simulink library "lib_Convection_LamIntFlwVarShapes"  (R2015a)
settings: Solver=ode45  StartTime=0.0  StopTime=10.0  RelTol=1e-3
libraries: simulink x5, lib_GenTools_MinMax x1
settings Model: Creator=jlkratz  LastModifiedBy=jlkratz

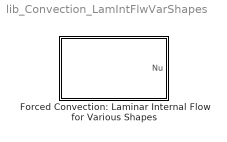
== system lib_Convection_LamIntFlwVarShapes ==
  Forced Convection: Laminar Internal Flow for Various Shapes : Subsystem  mask(TSAT: Laminar Flow for Various Shaped Tubes){Shape_M=Circle, IsothermOrIsoflux_M=Isothermal, FinOrInf_M=Finite Aspect Ratio, boa_M=1, HeatBothOrInsulateOne_M=Both sides heated}
      mask prompts: Shape_M "Shape_M - Cross-section shape"; IsothermOrIsoflux_M "IsothermOrIsoflux_M - Check for isothermal surfaces, unchecked for isoflux surfaces"; boa_M "boa_M - Aspect ratio of the rectangular cross-section (b/a) where b is the longer side"
      mask help:
      | This block provides the Nusselt number for fully developed laminar flow within tubes of different cross-sections. Options include circular, rectangular, and triangular cross-sections with isothermal and isoflux surfaces. In the case of rectangular flow paths the scenario of an infinite aspect ratio flow path is considered. This situation has options for when both sides of the flow path are heated and when one side is heated and the other is insulated. Note that when using the Nusselt number to calculate the convective heat transfer coefficient, the hydraulic diameter should be used.
      |
      | See the block help menu for more details.
      mask Help: web(which('Convection_TSAT_LamIntFlwVarShapes.html'),'-helpbrowser')
      mask TypeOptions Shape_M: Circle | Rectangle | Equilateral Triangle
      mask Callback Shape_M:
      | sel1 = get_param(gcb,'Shape_M');
      | sel2 = get_param(gcb,'FinOrInf_M');
      | if sel1(1) == 'R'
      |     MSK_SEC_Enables3_TSAT('on',[3],'en')
      |     if sel2(1) == 'F'
      |         MSK_SEC_Enables3_TSAT('on',[4],'en')
      |     elseif sel2(1) == 'I'
      |         MSK_SEC_Enables3_TSAT('on',[5],'en')
      |     end
      | else
      |     MSK_SEC_Enables3_TSAT('on',[3 4 5],'dis')
      | end
      | clear sel
      mask TypeOptions IsothermOrIsoflux_M: Isothermal | Isoflux
      mask TypeOptions FinOrInf_M: Finite Aspect Ratio | Infinite Aspect Ratio
      mask Callback FinOrInf_M:
      | sel1 = get_param(gcb,'FinOrInf_M');
      | sel2 = get_param(gcb,'Shape_M');
      | if sel2(1) == 'R'
      |     if sel1(1) == 'F'
      |         MSK_SEC_Enables3_TSAT('on',[4],'en')
      |         MSK_SEC_Enables3_TSAT('on',[5],'dis')
      |     elseif sel1(1) == 'I'
      |         MSK_SEC_Enables3_TSAT('on',[5],'en')
      |         MSK_SEC_Enables3_TSAT('on',[4],'dis')
      |     end
      | end
      | clear sel1 sel2
      mask TypeOptions HeatBothOrInsulateOne_M: Both sides heated | One side heated and the other insulated
      mask DialogControl Container3 Prompt: Applies to All
      mask DialogControl Container4 Prompt: Applies to Rectangles Only
      mask DialogControl Container5 Prompt: Finite Aspect Ratio Rectangles
      mask DialogControl Container6 Prompt: Infinite Aspect Ratio Rectangles

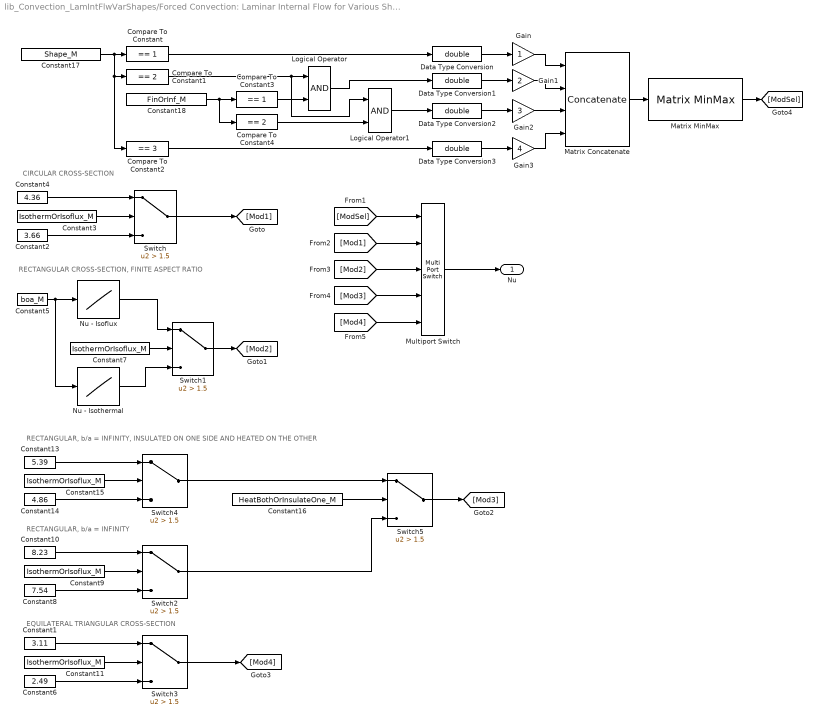
== system lib_Convection_LamIntFlwVarShapes/Forced Convection: Laminar Internal Flow for Various Shapes ==
  note: RECTANGULAR, b/a = INFINITY, INSULATED ON ONE SIDE AND HEATED ON THE OTHER
  note: EQUILATERAL TRIANGULAR CROSS-SECTION
  note: CIRCULAR CROSS-SECTION
  note: RECTANGULAR CROSS-SECTION, FINITE ASPECT RATIO
  note: RECTANGULAR, b/a = INFINITY
  Compare To Constant : simulink/Logic and Bit Operations/Compare To Constant  relop===  const=1  OutDataTypeStr=boolean
  Compare To Constant1 : simulink/Logic and Bit Operations/Compare To Constant  relop===  const=2  OutDataTypeStr=boolean
  Compare To Constant2 : simulink/Logic and Bit Operations/Compare To Constant  relop===  const=3  OutDataTypeStr=boolean
  Compare To Constant3 : simulink/Logic and Bit Operations/Compare To Constant  relop===  const=1  OutDataTypeStr=boolean
  Compare To Constant4 : simulink/Logic and Bit Operations/Compare To Constant  relop===  const=2  OutDataTypeStr=boolean
  Constant1 : Constant  Value=3.11
  Constant10 : Constant  Value=8.23
  Constant{3,7,9,11,15} (5 alike) : Constant  Value=IsothermOrIsoflux_M
  Constant13 : Constant  Value=5.39
  Constant14 : Constant  Value=4.86
  Constant16 : Constant  Value=HeatBothOrInsulateOne_M
  Constant17 : Constant  Value=Shape_M
  Constant18 : Constant  Value=FinOrInf_M
  Constant2 : Constant  Value=3.66
  Constant4 : Constant  Value=4.36
  Constant5 : Constant  Value=boa_M
  Constant6 : Constant  Value=2.49
  Constant8 : Constant  Value=7.54
  Data Type Conversion{,1..3} (4 alike) : DataTypeConversion  OutDataTypeStr=double
  Gain : Gain
  Gain1 : Gain  Gain=2
  Gain2 : Gain  Gain=3
  Gain3 : Gain  Gain=4
  Logical Operator : Logic  AllPortsSameDT=off  OutDataTypeStr=boolean
  Logical Operator1 : Logic  AllPortsSameDT=off  OutDataTypeStr=boolean
  Matrix Concatenate : Concatenate  NumInputs=4  Mode=Multidimensional array  ConcatenateDimension=2
  Matrix MinMax : lib_GenTools_MinMax/Matrix MinMax  rows_M=on  cols_M=off  all_M=off  minmax_M=off  BN_M=gcb
  Multiport Switch : MultiPortSwitch  Inputs=4
  Nu - Isoflux : Lookup_n-D  NumberOfTableDimensions=1  BreakpointsForDimension1=[1 1.43 1.75 2 2.5 3 3.5 4 4.5 5 6 7 8 9 10 12 15 18 20 23 25 28 32 40 47 100]  Table=[3.6100 3.7300 3.9349 4.1200 4.4722 4.7900 5.0760 5.3300 5.5517 5.7441 6.0556 6.2944 6.4900 6.6673 6.8316 7.1235 7.4767 7.7406 7.8735 8.0187 8.0851 8.1493 8.1899 8.2201 8.2300 8.2300]  InternalRulePriority=Speed  RndMeth=Simplest  InputSameDT=on
  Nu - Isothermal : Lookup_n-D  NumberOfTableDimensions=1  BreakpointsForDimension1=[1 1.43 1.75 2 2.5 3 3.5 4 4.5 5 6 7 8 9 10 12 15 18 20 23 25 28 32 40 45 100]  Table=[2.9800 3.0800 3.2418 3.3900 3.6839 3.9600 4.2124 4.4400 4.6435 4.8252 5.1332 5.3845 5.6000 5.7968 5.9790 6.3016 6.6904 6.9793 7.1243 7.2825 7.3553 7.4276 7.4800 7.5300 7.5400 7.5400]  InternalRulePriority=Speed  RndMeth=Simplest  InputSameDT=on
  Switch{,1..5} (6 alike) : Switch  Criteria=u2 > Threshold  Threshold=1.5
  Nu : Outport
  wires:
  Gain3/1 -> Matrix Concatenate/4
  Gain2/1 -> Matrix Concatenate/3
  Gain1/1 -> Matrix Concatenate/2
  Gain/1 -> Matrix Concatenate/1
  Matrix Concatenate/1 -> Matrix MinMax/1
  Matrix MinMax/1 -> [ModSel]
  Data Type Conversion3/1 -> Gain3/1
  Data Type Conversion2/1 -> Gain2/1
  Data Type Conversion1/1 -> Gain1/1
  Data Type Conversion/1 -> Gain/1
  Compare To Constant2/1 -> Data Type Conversion3/1
  Logical Operator1/1 -> Data Type Conversion2/1
  Logical Operator/1 -> Data Type Conversion1/1
  Compare To Constant/1 -> Data Type Conversion/1
  Compare To Constant4/1 -> Logical Operator1/2
  Compare To Constant3/1 -> Logical Operator/2
  Compare To Constant1/1 -> Logical Operator/1, Logical Operator1/1
  Constant18/1 -> Compare To Constant3/1, Compare To Constant4/1
  Constant17/1 -> Compare To Constant/1, Compare To Constant1/1, Compare To Constant2/1
  Constant16/1 -> Switch5/2
  Switch4/1 -> Switch5/1
  Switch2/1 -> Switch5/3
  Switch5/1 -> [Mod3]
  Constant15/1 -> Switch4/2
  Constant13/1 -> Switch4/1
  Constant14/1 -> Switch4/3
  [ModSel] -> Multiport Switch/1
  [Mod3] -> Multiport Switch/4
  [Mod2] -> Multiport Switch/3
  Multiport Switch/1 -> Nu/1
  Switch3/1 -> [Mod4]
  [Mod4] -> Multiport Switch/5
  Constant1/1 -> Switch3/1
  Constant9/1 -> Switch2/2
  Constant10/1 -> Switch2/1
  [Mod1] -> Multiport Switch/2
  Switch/1 -> [Mod1]
  Constant8/1 -> Switch2/3
  Switch1/1 -> [Mod2]
  Constant2/1 -> Switch/3
  Constant6/1 -> Switch3/3
  Constant11/1 -> Switch3/2
  Nu - Isoflux/1 -> Switch1/1
  Nu - Isothermal/1 -> Switch1/3
  Constant7/1 -> Switch1/2
  Constant4/1 -> Switch/1
  Constant3/1 -> Switch/2
  Constant5/1 -> Nu - Isothermal/1, Nu - Isoflux/1
